simulink model "lateral_autopilot_full_2g"  (R2016b)
settings: Solver=VariableStepAuto  StartTime=0.0  StopTime=t_end  RelTol=1e-3
values from neighbouring files (symbols this model uses):
  A = [ -0.322 0.052 0.028 -1.12 0.002 ... (first row only)    [parameters_longitudal_autopilot.m]
  B = [ 0 0 0 0 10]'    [parameters_longitudal_autopilot.m]
  C = [0 0 0 1 0 ... (first row only)    [parameters_longitudal_autopilot.m]
  D = [0 0 0 0]'    [parameters_longitudal_autopilot.m]
  d = 2*deg2rad    [run_task_2f.m]    (also in run_task_2g.m = 10*deg2rad)
  delta_a_max = 25*deg2rad    (= 0.436332312999)    [parameters_longitudal_autopilot.m]
  g = 9.81    [parameters_longitudal_autopilot.m]
  k_d_phi = (2*zeta_phi*omega_n_phi - a_phi_1) / a_phi_2    [parameters_longitudal_autopilot.m]
  k_i_chi = omega_n_chi^2*V_g/g    [parameters_longitudal_autopilot.m]
  k_i_phi = 0    [parameters_longitudal_autopilot.m]
  k_p_chi = 3.75    [parameters_longitudal_autopilot.m]
  k_p_phi = sign(a_phi_2)*delta_a_max /e_phi_max    [parameters_longitudal_autopilot.m]
  V_g = 637/3.6    (= 176.944444444)    [parameters_longitudal_autopilot.m]
undefined symbols (not defined in the file or in its folder): integrator_error_limit
settings Model: Creator=EllaLovise  LastModifiedBy=EllaLovise

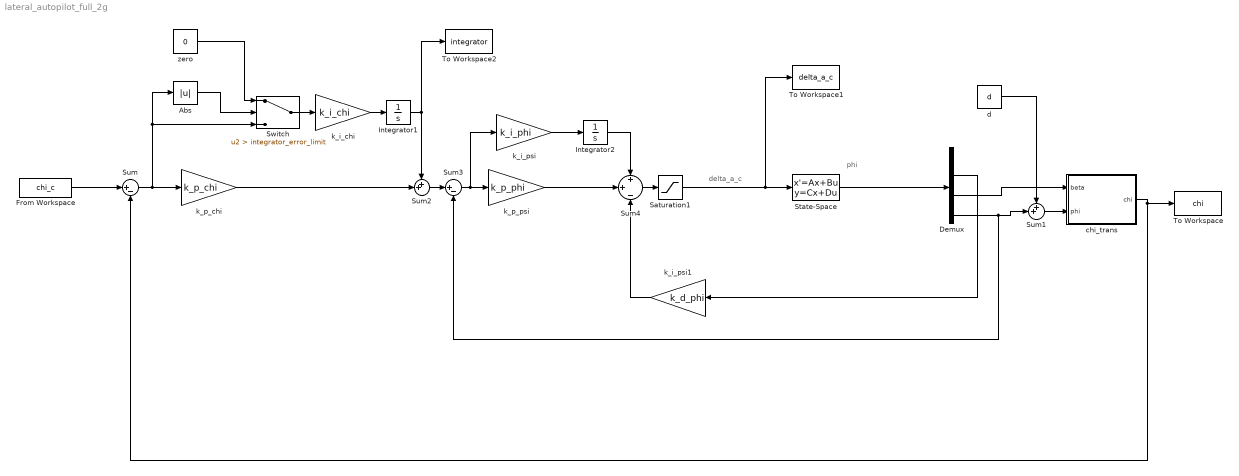
== system lateral_autopilot_full_2g ==
  note: phi
  note: delta_a_c
  Abs : Abs  ZeroCross=off
  Demux : Demux
  From Workspace : FromWorkspace  VariableName=chi_c  OutputAfterFinalValue=Holding final value
  Integrator1 : Integrator
  Integrator2 : Integrator
  Saturation1 : Saturate  UpperLimit=delta_a_max  LowerLimit=-1*delta_a_max
  State-Space : StateSpace  A=A  B=B  C=C  D=D  X0=0
  Sum : Sum  Inputs=|+-
  Sum1 : Sum  Inputs=++|
  Sum2 : Sum  Inputs=++|
  Sum3 : Sum  Inputs=|+-
  Sum4 : Sum  Inputs=+|+|-
  Switch : Switch  Criteria=u2 > Threshold  Threshold=integrator_error_limit
  To Workspace : ToWorkspace  VariableName=chi  SaveFormat=Structure With Time  SampleTime=-1
  To Workspace1 : ToWorkspace  VariableName=delta_a_c  SaveFormat=Structure With Time  SampleTime=-1
  To Workspace2 : ToWorkspace  VariableName=integrator  SaveFormat=Structure With Time  SampleTime=-1
  chi_trans : Subsystem
  d : Constant  Value=d
  k_i_chi : Gain  Gain=k_i_chi
  k_i_psi : Gain  Gain=k_i_phi
  k_i_psi1 : Gain  Gain=k_d_phi
  k_p_chi : Gain  Gain=k_p_chi
  k_p_psi : Gain  Gain=k_p_phi
  zero : Constant  Value=0
  wires:
  From Workspace/1 -> Sum/1
  Sum/1 -> k_p_chi/1, Abs/1, Switch/3
  k_p_chi/1 -> Sum2/2
  Sum2/1 -> Sum3/1
  Sum3/1 -> k_i_psi/1, k_p_psi/1
  k_i_psi/1 -> Integrator2/1
  chi_trans/1(chi) -> Sum/2, To Workspace/1
  k_i_chi/1 -> Integrator1/1
  k_p_psi/1 -> Sum4/2
  k_i_psi1/1 -> Sum4/3
  Demux/4 -> Sum3/2, Sum1/2
  Demux/3 -> chi_trans/1(beta)
  Demux/2 -> k_i_psi1/1
  Saturation1/1 -> To Workspace1/1, State-Space/1
  Sum4/1 -> Saturation1/1
  State-Space/1 -> Demux/1
  d/1 -> Sum1/1
  Integrator2/1 -> Sum4/1
  Integrator1/1 -> Sum2/1, To Workspace2/1
  Sum1/1 -> chi_trans/2(phi)
  Abs/1 -> Switch/2
  Switch/1 -> k_i_chi/1
  zero/1 -> Switch/1

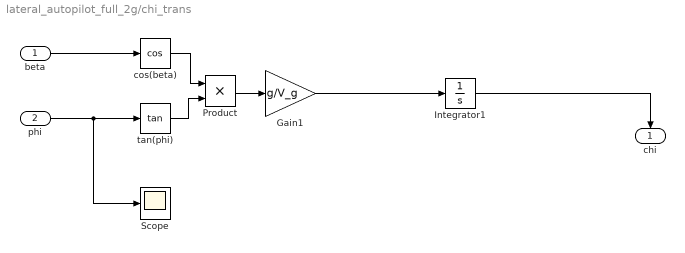
== system lateral_autopilot_full_2g/chi_trans ==
  beta : Inport
  phi : Inport  Port=2
  Gain1 : Gain  Gain=g/V_g
  Integrator1 : Integrator
  Product : Product
  Scope : Scope
  cos(beta) : Trigonometry  Operator=cos
  tan(phi) : Trigonometry  Operator=tan
  chi : Outport
  wires:
  phi/1 -> Scope/1, tan(phi)/1
  Integrator1/1 -> chi/1
  beta/1 -> cos(beta)/1
  tan(phi)/1 -> Product/2
  Product/1 -> Gain1/1
  cos(beta)/1 -> Product/1
  Gain1/1 -> Integrator1/1
